simulink model "test_direct"  (R2024a)
settings: Solver=VariableStepAuto  StartTime=0.0  StopTime=40  RelTol=1e-3
libraries: neural x733, simulink x4
(part 25 of 35)

== system test_direct/Function Fitting Neural Network5/Layer 2/LW{2,1} ==
  "ad{2,1}" : Inport  PortDimensions=20
      mask Display: e = 0.06;c1 = [120 230 180]/255;c2 = ([120 230 180]+0)/(256+128);c3 = ([120 230 180]+128)/(256+128);patch([0 1 1 0],[0 0 1 1],c1);patch([0 1 1 1-e 1-e 0+e],[0 0 1 1-e 0+e 0+e],c2);patch([0 0 1 1-e 0+e 0+e],[0 1 1 1-e 1-e 0+e],c3);plot([0 1 1 0 0],[0 0 1 1 0]);
  "IW{2,1}(1,:)'" : Constant  Value=[-0.579046845479741278950314153917133808135986328125;-0.366332767141648307784862481639720499515533447265625;0.00791926397557877158328576427948064520023763179779052734375;0.355333435528304930617338186493725515902042388916015625;-0.19644275811117173358155696405447088181972503662109375;0.254735292145369107696950550234760157763957977294921875;0.36445816412065534795061694239848293364048004150390625;0.0304633669830193902494652746781866881065070629119873046875;0.74146026581714241654452735019731335341930389404296875;-0.0411865383465370438198505098625901155173778533935546875;0.10211270720633357222961734578348114155232906341552734375;0.1094855228463350871326298374697216786444187164306640625;1.093274183178303271546383257373236119747161865234375;-0.099686376669609499945323705105693079531192779541015625;-0.1438151389707562899378245901971240527927875518798828125;0.1476459310225679832928591395102557726204395294189453125;0.02646611700207172901411212251332472078502178192138671875;-0.42917127450968506341411057292134501039981842041015625;-0.184180448452047673679743411412346176803112030029296875;-0.0920595225436459940748790131692658178508281707763671875]
      mask Display: e = 0.06;c1 = [120 150 230]/255;c2 = ([120 150 230]+0)/383;c3 = ([120 150 230]+128)/383;patch([0 1 1 0],[0 0 1 1],c1);patch([0 1 1 1-e 1-e 0+e],[0 0 1 1-e 0+e 0+e],c2);patch([0 0 1 1-e 0+e 0+e],[0 1 1 1-e 1-e 0+e],c3);plot([0 1 1 0 0],[0 0 1 1 0]);disp('weights');
  "IW{2,1}(10,:)'" : Constant  Value=[0.45106523314206070640608459143550135195255279541015625;-0.006484688981325256902643605627645229105837643146514892578125;-0.600418159129877171409361835685558617115020751953125;0.59913844375957359122963907793746329843997955322265625;-0.76623092060152242499526664687437005341053009033203125;0.234260916721591883060682448558509349822998046875;0.7292760586627295982253826878149993717670440673828125;-0.449833710963811750360719088348560035228729248046875;0.3274752254953769980971856057294644415378570556640625;-0.47734563271799601569256310540367849171161651611328125;1.2532004567650962822966675958014093339443206787109375;-0.232482810204428125278042216450558044016361236572265625;-0.51335343850787673591895554636721499264240264892578125;0.01036668286886731869811395512215312919579446315765380859375;-0.0277386185034186084907847913427758612670004367828369140625;-0.049524443823777804241093036807797034271061420440673828125;0.02041516786832299479303998168688849546015262603759765625;0.013914717500251472248606887660571373999118804931640625;-0.041074885648775254221032326995555195026099681854248046875;-0.07560051804477367631829309857494081370532512664794921875]
      mask Display: e = 0.06;c1 = [120 150 230]/255;c2 = ([120 150 230]+0)/383;c3 = ([120 150 230]+128)/383;patch([0 1 1 0],[0 0 1 1],c1);patch([0 1 1 1-e 1-e 0+e],[0 0 1 1-e 0+e 0+e],c2);patch([0 0 1 1-e 0+e 0+e],[0 1 1 1-e 1-e 0+e],c3);plot([0 1 1 0 0],[0 0 1 1 0]);disp('weights');
  "IW{2,1}(2,:)'" : Constant  Value=[0.246046120338173024411076994510949589312076568603515625;-0.44416355549470665220468390543828718364238739013671875;-0.241828085176459761651557300865533761680126190185546875;0.048803101340167388821900118500707321800291538238525390625;0.2146749034455693594392045042695826850831508636474609375;-0.214628473377201867133834412015858106315135955810546875;0.304852751461086535211819636970176361501216888427734375;-0.26261872451235446224160341444076038897037506103515625;-0.37883423077533040501663208488025702536106109619140625;-0.262512916868190782082592704682610929012298583984375;-0.302067842690707577535391692435950972139835357666015625;-0.2059116523634101358908310430706478655338287353515625;0.277348751006312621569804832688532769680023193359375;-0.0667686637669950566742471664838376455008983612060546875;0.1551576203481833393649225172339356504380702972412109375;-0.156817869861261283137565669676405377686023712158203125;-0.64778006144449074010793765410198830068111419677734375;0.190002056867068558343447648439905606210231781005859375;0.3183559563991422702855516035924665629863739013671875;-0.65511604508801413171426020198850892484188079833984375]
      mask Display: e = 0.06;c1 = [120 150 230]/255;c2 = ([120 150 230]+0)/383;c3 = ([120 150 230]+128)/383;patch([0 1 1 0],[0 0 1 1],c1);patch([0 1 1 1-e 1-e 0+e],[0 0 1 1-e 0+e 0+e],c2);patch([0 0 1 1-e 0+e 0+e],[0 1 1 1-e 1-e 0+e],c3);plot([0 1 1 0 0],[0 0 1 1 0]);disp('weights');
  "IW{2,1}(3,:)'" : Constant  Value=[-0.352192261129181949375066551510826684534549713134765625;0.293665677168537087027289089746773242950439453125;-0.315518300729069889332123466374468989670276641845703125;-0.46790601172040224842163524954230524599552154541015625;0.0647169840392622652824883289213175885379314422607421875;-0.22641417805884866965016044559888541698455810546875;-0.421662956096390650895244789353455416858196258544921875;0.09447283223856751954716770569575601257383823394775390625;0.94313894621172511545381667019682936370372772216796875;0.182850302879195958372093855359707958996295928955078125;-0.2185526225368461805675934783721459098160266876220703125;-0.00908050016434655722641355879432012443430721759796142578125;0.7216056503661600896037953134509734809398651123046875;0.0604873719582102176151039429896627552807331085205078125;0.092237612451127104495895991931320168077945709228515625;-0.1472698116716875116338769657886587083339691162109375;0.0003899457974927842611283235196850682768854312598705291748046875;-0.071899880019338391345939953680499456822872161865234375;0.058786601922839187839286978487507440149784088134765625;0.07787533088066123099224569159559905529022216796875]
      mask Display: e = 0.06;c1 = [120 150 230]/255;c2 = ([120 150 230]+0)/383;c3 = ([120 150 230]+128)/383;patch([0 1 1 0],[0 0 1 1],c1);patch([0 1 1 1-e 1-e 0+e],[0 0 1 1-e 0+e 0+e],c2);patch([0 0 1 1-e 0+e 0+e],[0 1 1 1-e 1-e 0+e],c3);plot([0 1 1 0 0],[0 0 1 1 0]);disp('weights');
  "IW{2,1}(4,:)'" : Constant  Value=[-0.11038535014864879479912218585013761185109615325927734375;0.069052015333759708681782285566441714763641357421875;0.278344839855194148281469779249164275825023651123046875;-0.0429139321375657523116586844480480067431926727294921875;-0.14827093883976172339345112050068564713001251220703125;0.18100889775099648915102079627104103565216064453125;0.2070239482488422655404036731852102093398571014404296875;-0.1063017601653035992814722021648776717483997344970703125;-1.318163989884748144021386906388215720653533935546875;-0.098737455922967232169185081147588789463043212890625;0.214362322162434171257672232968616299331188201904296875;-0.03863337852201731426049491346930153667926788330078125;-0.588383198236690940774451519246213138103485107421875;-0.0272585835270687422415836209665940259583294391632080078125;0.000514366209257961369723244349216884074849076569080352783203125;0.054695929844052380841556981749818078242242336273193359375;-0.020553438564307725811008964456050307489931583404541015625;-0.468404405522319711163703459533280692994594573974609375;-0.02550599518226213946459068893091171048581600189208984375;-0.1348161547458721631898015402839519083499908447265625]
      mask Display: e = 0.06;c1 = [120 150 230]/255;c2 = ([120 150 230]+0)/383;c3 = ([120 150 230]+128)/383;patch([0 1 1 0],[0 0 1 1],c1);patch([0 1 1 1-e 1-e 0+e],[0 0 1 1-e 0+e 0+e],c2);patch([0 0 1 1-e 0+e 0+e],[0 1 1 1-e 1-e 0+e],c3);plot([0 1 1 0 0],[0 0 1 1 0]);disp('weights');
  "IW{2,1}(5,:)'" : Constant  Value=[0.7023428356000043226714524280396290123462677001953125;-0.184530133447649624667263879018719308078289031982421875;-0.1973243620284037824763601065569673664867877960205078125;0.352442802646694752777278836219920776784420013427734375;0.06548962322746569586495724024644005112349987030029296875;-0.538534813181375415780394178000278770923614501953125;0.027054454061479417392721558144330629147589206695556640625;0.4849622461151159580339253807323984801769256591796875;0.3562846230078176024136382693541236221790313720703125;0.2082065434670395120964059287871350534260272979736328125;0.647547883714221228501628502272069454193115234375;0.247394932810874268458434244166710413992404937744140625;-0.80148602251719880396052531068562529981136322021484375;0.0224490783621045415785477672443448682315647602081298828125;0.0869778231743936480757639628791366703808307647705078125;-0.2207666330910662277897671401660772971808910369873046875;-0.017685957506404927086496314814212382771074771881103515625;-0.34856979109160557417368409005575813353061676025390625;0.060254870992509833305117439294917858205735683441162109375;0.430945889886455102413265194627456367015838623046875]
      mask Display: e = 0.06;c1 = [120 150 230]/255;c2 = ([120 150 230]+0)/383;c3 = ([120 150 230]+128)/383;patch([0 1 1 0],[0 0 1 1],c1);patch([0 1 1 1-e 1-e 0+e],[0 0 1 1-e 0+e 0+e],c2);patch([0 0 1 1-e 0+e 0+e],[0 1 1 1-e 1-e 0+e],c3);plot([0 1 1 0 0],[0 0 1 1 0]);disp('weights');
  "IW{2,1}(6,:)'" : Constant  Value=[0.4224089115452738241174301947467029094696044921875;0.440056808161991386274536353084840811789035797119140625;-0.11419472374626714328282872656927793286740779876708984375;0.57575449411118595488545679472736082971096038818359375;-0.2331470229256961401720360527178854681551456451416015625;-0.423016524638085422704847360364510677754878997802734375;1.363489995339575155952616114518605172634124755859375;-1.0868187458133322653708319194265641272068023681640625;-0.10913236701853497312431073851257679052650928497314453125;0.799982620513981945720161093049682676792144775390625;-0.182307650456612180267512712816824205219745635986328125;0.37545487088480145043689617523341439664363861083984375;0.41570000943437579454808883383520878851413726806640625;0.023541045860106489528984496928387670777738094329833984375;0.473684260454336258927554581532604061067104339599609375;1.2657571479447373707927226860192604362964630126953125;-0.1829983548740201637627933450858108699321746826171875;-0.221247927654384113349550489147077314555644989013671875;-0.367143898363431142595203482414945028722286224365234375;0.0019581555874889507683211942179468678659759461879730224609375]
      mask Display: e = 0.06;c1 = [120 150 230]/255;c2 = ([120 150 230]+0)/383;c3 = ([120 150 230]+128)/383;patch([0 1 1 0],[0 0 1 1],c1);patch([0 1 1 1-e 1-e 0+e],[0 0 1 1-e 0+e 0+e],c2);patch([0 0 1 1-e 0+e 0+e],[0 1 1 1-e 1-e 0+e],c3);plot([0 1 1 0 0],[0 0 1 1 0]);disp('weights');
  "IW{2,1}(7,:)'" : Constant  Value=[0.85279025027125465729938014192157424986362457275390625;0.08683805962927020061226102143336902372539043426513671875;-0.1673040176973877024568793103753705509006977081298828125;0.184731321925173885833970643943757750093936920166015625;0.7682354316165156404849767568521201610565185546875;-0.1796643086082986007223638580398983322083950042724609375;0.521167175396772375250975528615526854991912841796875;0.297359432301631476658343444796628318727016448974609375;0.99940927153345715527876791384187527000904083251953125;-0.4141002194910043954223510809242725372314453125;0.277484240839730500471915775051456876099109649658203125;0.3502208837605882418841929393238388001918792724609375;-0.51455921650667202360551755191409029066562652587890625;-0.022741456932024471659925524136269814334809780120849609375;0.270467721739372113365362793047097511589527130126953125;-0.08357141079773365566207843357915407977998256683349609375;-0.1332513992108804445901881763347773812711238861083984375;0.0696241608697020508689234929988742806017398834228515625;0.311943119438749472127625494977110065519809722900390625;-0.032764834535114299718383534809618140570819377899169921875]
      mask Display: e = 0.06;c1 = [120 150 230]/255;c2 = ([120 150 230]+0)/383;c3 = ([120 150 230]+128)/383;patch([0 1 1 0],[0 0 1 1],c1);patch([0 1 1 1-e 1-e 0+e],[0 0 1 1-e 0+e 0+e],c2);patch([0 0 1 1-e 0+e 0+e],[0 1 1 1-e 1-e 0+e],c3);plot([0 1 1 0 0],[0 0 1 1 0]);disp('weights');
  "IW{2,1}(8,:)'" : Constant  Value=[0.498452840354915716059025498907431028783321380615234375;0.366558574940812842424264772489550523459911346435546875;-0.1510456402745621318217672524042427539825439453125;-0.0769269745328168552678249625387252308428287506103515625;0.3004215881244201025168649721308611333370208740234375;-0.490819816489340199350266402689157985150814056396484375;0.1364661808556923150437256708755739964544773101806640625;0.384791567617603524897873512600199319422245025634765625;0.7867187025807071965033401284017600119113922119140625;-0.6146433979166905370306039912975393235683441162109375;0.497314382965974022265953635724144987761974334716796875;-0.08779484862380086684918722994552808813750743865966796875;-0.08995292924666446754411452957356232218444347381591796875;-0.07126163880156348440220170914471964351832866668701171875;-0.756117230801268913609192168223671615123748779296875;0.0225922316589895998129033927170894457958638668060302734375;0.313500674283847702294991677263169549405574798583984375;0.11989233760044448739989775276626460254192352294921875;-0.18563408446150686526010531451902352273464202880859375;-0.050881810495495095880702507429305114783346652984619140625]
      mask Display: e = 0.06;c1 = [120 150 230]/255;c2 = ([120 150 230]+0)/383;c3 = ([120 150 230]+128)/383;patch([0 1 1 0],[0 0 1 1],c1);patch([0 1 1 1-e 1-e 0+e],[0 0 1 1-e 0+e 0+e],c2);patch([0 0 1 1-e 0+e 0+e],[0 1 1 1-e 1-e 0+e],c3);plot([0 1 1 0 0],[0 0 1 1 0]);disp('weights');
  "IW{2,1}(9,:)'" : Constant  Value=[0.290579186072249751049412225256673991680145263671875;0.366662252183763082147294198875897563993930816650390625;0.1440875193407215870688986569803091697394847869873046875;-0.0302403581180806131645244505534719792194664478302001953125;0.100950277691890966114129923880682326853275299072265625;0.1381393716982420583061497154631069861352443695068359375;0.331727150444919127725285079577588476240634918212890625;-0.4425342659789885946253207293921150267124176025390625;-0.023796097376492665598224363066037767566740512847900390625;0.25120426572081366867195129088941030204296112060546875;-0.287894666419527600620398288810974918305873870849609375;-0.157619878708374294706828777634655125439167022705078125;-0.6348198907290776293876888303202576935291290283203125;0.10107959034423912025868474984235945157706737518310546875;0.6616827948368395606593139746109955012798309326171875;-0.487640617460125491700040356590761803090572357177734375;-0.380966735137811596256796065063099376857280731201171875;0.1969944624768071583797990342645789496600627899169921875;0.491439123097786201288528218356077559292316436767578125;-0.481116141212482417710560866908053867518901824951171875]
      mask Display: e = 0.06;c1 = [120 150 230]/255;c2 = ([120 150 230]+0)/383;c3 = ([120 150 230]+128)/383;patch([0 1 1 0],[0 0 1 1],c1);patch([0 1 1 1-e 1-e 0+e],[0 0 1 1-e 0+e 0+e],c2);patch([0 0 1 1-e 0+e 0+e],[0 1 1 1-e 1-e 0+e],c3);plot([0 1 1 0 0],[0 0 1 1 0]);disp('weights');
  Mux : Mux  Inputs=10
      mask Display: e = 0.06;c1 = [120 150 230]/255;c2 = ([120 150 230]+0)/383;c3 = ([120 150 230]+128)/383;patch([0 1 1 0],[0 0 1 1],c1);patch([0 1 1 1-e 1-e 0+e],[0 0 1 1-e 0+e 0+e],c2);patch([0 0 1 1-e 0+e 0+e],[0 1 1 1-e 1-e 0+e],c3);plot([0 1 1 0 0],[0 0 1 1 0]);disp('Mux');
  dotprod{1..10} (10 alike) : neural/Weight Functions/dotprod
  "lz{2,1}" : Outport
      mask Display: e = 0.06;c1 = [120 230 180]/255;c2 = ([120 230 180]+0)/(256+128);c3 = ([120 230 180]+128)/(256+128);patch([0 1 1 0],[0 0 1 1],c1);patch([0 1 1 1-e 1-e 0+e],[0 0 1 1-e 0+e 0+e],c2);patch([0 0 1 1-e 0+e 0+e],[0 1 1 1-e 1-e 0+e],c3);plot([0 1 1 0 0],[0 0 1 1 0]);
  wires:
  "IW{2,1}(1,:)'"/1 -> dotprod1/1
  "ad{2,1}"/1 -> dotprod1/2, dotprod2/2, dotprod3/2, dotprod4/2, dotprod5/2, dotprod6/2, dotprod7/2, dotprod8/2, dotprod9/2, dotprod10/2
  dotprod1/1 -> Mux/1
  "IW{2,1}(2,:)'"/1 -> dotprod2/1
  dotprod2/1 -> Mux/2
  "IW{2,1}(3,:)'"/1 -> dotprod3/1
  dotprod3/1 -> Mux/3
  "IW{2,1}(4,:)'"/1 -> dotprod4/1
  dotprod4/1 -> Mux/4
  "IW{2,1}(5,:)'"/1 -> dotprod5/1
  dotprod5/1 -> Mux/5
  "IW{2,1}(6,:)'"/1 -> dotprod6/1
  dotprod6/1 -> Mux/6
  "IW{2,1}(7,:)'"/1 -> dotprod7/1
  dotprod7/1 -> Mux/7
  "IW{2,1}(8,:)'"/1 -> dotprod8/1
  dotprod8/1 -> Mux/8
  "IW{2,1}(9,:)'"/1 -> dotprod9/1
  dotprod9/1 -> Mux/9
  "IW{2,1}(10,:)'"/1 -> dotprod10/1
  dotprod10/1 -> Mux/10
  Mux/1 -> "lz{2,1}"/1

== system test_direct/Function Fitting Neural Network5/Layer 3/Delays 1 ==
  "p{3}" : Inport  PortDimensions=10
      mask Display: e = 0.06;c1 = [120 230 180]/255;c2 = ([120 230 180]+0)/(256+128);c3 = ([120 230 180]+128)/(256+128);patch([0 1 1 0],[0 0 1 1],c1);patch([0 1 1 1-e 1-e 0+e],[0 0 1 1-e 0+e 0+e],c2);patch([0 0 1 1-e 0+e 0+e],[0 1 1 1-e 1-e 0+e],c3);plot([0 1 1 0 0],[0 0 1 1 0]);
  mux : Mux  Inputs=1
      mask Display: e = 0.06;c1 = [120 150 230]/255;c2 = ([120 150 230]+0)/383;c3 = ([120 150 230]+128)/383;patch([0 1 1 0],[0 0 1 1],c1);patch([0 1 1 1-e 1-e 0+e],[0 0 1 1-e 0+e 0+e],c2);patch([0 0 1 1-e 0+e 0+e],[0 1 1 1-e 1-e 0+e],c3);plot([0 1 1 0 0],[0 0 1 1 0]);disp('Mux')
  "pd{3,2}" : Outport
      mask Display: e = 0.06;c1 = [120 230 180]/255;c2 = ([120 230 180]+0)/(256+128);c3 = ([120 230 180]+128)/(256+128);patch([0 1 1 0],[0 0 1 1],c1);patch([0 1 1 1-e 1-e 0+e],[0 0 1 1-e 0+e 0+e],c2);patch([0 0 1 1-e 0+e 0+e],[0 1 1 1-e 1-e 0+e],c3);plot([0 1 1 0 0],[0 0 1 1 0]);
  wires:
  "p{3}"/1 -> mux/1
  mux/1 -> "pd{3,2}"/1

== system test_direct/Function Fitting Neural Network5/Layer 3/LW{3,2} ==
  "ad{3,2}" : Inport  PortDimensions=10
      mask Display: e = 0.06;c1 = [120 230 180]/255;c2 = ([120 230 180]+0)/(256+128);c3 = ([120 230 180]+128)/(256+128);patch([0 1 1 0],[0 0 1 1],c1);patch([0 1 1 1-e 1-e 0+e],[0 0 1 1-e 0+e 0+e],c2);patch([0 0 1 1-e 0+e 0+e],[0 1 1 1-e 1-e 0+e],c3);plot([0 1 1 0 0],[0 0 1 1 0]);
  "IW{3,2}(1,:)'" : Constant  Value=[0.79370873300215050161199314970872364938259124755859375;-0.3200226311081910690603535840637050569057464599609375;1.2061996125942109348017083902959711849689483642578125;-1.5615997523335156671464574174024164676666259765625;-0.75490200592473011287353301668190397322177886962890625;-0.11063883079028712097535702696404769085347652435302734375;0.5845904369092311814171125661232508718967437744140625;0.04601777779405673285406663808316807262599468231201171875;-0.7115838685892506010333136146073229610919952392578125;-0.5017512522185627599213830762892030179500579833984375]
      mask Display: e = 0.06;c1 = [120 150 230]/255;c2 = ([120 150 230]+0)/383;c3 = ([120 150 230]+128)/383;patch([0 1 1 0],[0 0 1 1],c1);patch([0 1 1 1-e 1-e 0+e],[0 0 1 1-e 0+e 0+e],c2);patch([0 0 1 1-e 0+e 0+e],[0 1 1 1-e 1-e 0+e],c3);plot([0 1 1 0 0],[0 0 1 1 0]);disp('weights');
  "IW{3,2}(2,:)'" : Constant  Value=[-0.28960166204355208829923640223569236695766448974609375;-0.0252574701415183740238479259687665035016834735870361328125;-0.0958925927891242924072656705902772955596446990966796875;0.06445536465388544689059102665851241908967494964599609375;0.2594143192737743408571304826182313263416290283203125;0.16773287966872107990212725781020708382129669189453125;0.73734001878716337596841867707553319633007049560546875;0.10779251526925580362270551404435536824166774749755859375;0.03260513731556773098230195273572462610900402069091796875;0.97907124259663103060802313848398625850677490234375]
      mask Display: e = 0.06;c1 = [120 150 230]/255;c2 = ([120 150 230]+0)/383;c3 = ([120 150 230]+128)/383;patch([0 1 1 0],[0 0 1 1],c1);patch([0 1 1 1-e 1-e 0+e],[0 0 1 1-e 0+e 0+e],c2);patch([0 0 1 1-e 0+e 0+e],[0 1 1 1-e 1-e 0+e],c3);plot([0 1 1 0 0],[0 0 1 1 0]);disp('weights');
  Mux : Mux  Inputs=2
      mask Display: e = 0.06;c1 = [120 150 230]/255;c2 = ([120 150 230]+0)/383;c3 = ([120 150 230]+128)/383;patch([0 1 1 0],[0 0 1 1],c1);patch([0 1 1 1-e 1-e 0+e],[0 0 1 1-e 0+e 0+e],c2);patch([0 0 1 1-e 0+e 0+e],[0 1 1 1-e 1-e 0+e],c3);plot([0 1 1 0 0],[0 0 1 1 0]);disp('Mux');
  dotprod1 : neural/Weight Functions/dotprod
  dotprod2 : neural/Weight Functions/dotprod
  "lz{3,2}" : Outport
      mask Display: e = 0.06;c1 = [120 230 180]/255;c2 = ([120 230 180]+0)/(256+128);c3 = ([120 230 180]+128)/(256+128);patch([0 1 1 0],[0 0 1 1],c1);patch([0 1 1 1-e 1-e 0+e],[0 0 1 1-e 0+e 0+e],c2);patch([0 0 1 1-e 0+e 0+e],[0 1 1 1-e 1-e 0+e],c3);plot([0 1 1 0 0],[0 0 1 1 0]);
  wires:
  "IW{3,2}(1,:)'"/1 -> dotprod1/1
  "ad{3,2}"/1 -> dotprod1/2, dotprod2/2
  dotprod1/1 -> Mux/1
  "IW{3,2}(2,:)'"/1 -> dotprod2/1
  dotprod2/1 -> Mux/2
  Mux/1 -> "lz{3,2}"/1

== system test_direct/Function Fitting Neural Network6/Layer 1/Delays 1 ==
  "p{1}" : Inport  PortDimensions=8
      mask Display: e = 0.06;c1 = [120 230 180]/255;c2 = ([120 230 180]+0)/(256+128);c3 = ([120 230 180]+128)/(256+128);patch([0 1 1 0],[0 0 1 1],c1);patch([0 1 1 1-e 1-e 0+e],[0 0 1 1-e 0+e 0+e],c2);patch([0 0 1 1-e 0+e 0+e],[0 1 1 1-e 1-e 0+e],c3);plot([0 1 1 0 0],[0 0 1 1 0]);
  mux : Mux  Inputs=1
      mask Display: e = 0.06;c1 = [120 150 230]/255;c2 = ([120 150 230]+0)/383;c3 = ([120 150 230]+128)/383;patch([0 1 1 0],[0 0 1 1],c1);patch([0 1 1 1-e 1-e 0+e],[0 0 1 1-e 0+e 0+e],c2);patch([0 0 1 1-e 0+e 0+e],[0 1 1 1-e 1-e 0+e],c3);plot([0 1 1 0 0],[0 0 1 1 0]);disp('Mux')
  "pd{1,1}" : Outport
      mask Display: e = 0.06;c1 = [120 230 180]/255;c2 = ([120 230 180]+0)/(256+128);c3 = ([120 230 180]+128)/(256+128);patch([0 1 1 0],[0 0 1 1],c1);patch([0 1 1 1-e 1-e 0+e],[0 0 1 1-e 0+e 0+e],c2);patch([0 0 1 1-e 0+e 0+e],[0 1 1 1-e 1-e 0+e],c3);plot([0 1 1 0 0],[0 0 1 1 0]);
  wires:
  "p{1}"/1 -> mux/1
  mux/1 -> "pd{1,1}"/1

== system test_direct/Function Fitting Neural Network6/Layer 1/IW{1,1} ==
  "pd{1,1}" : Inport  PortDimensions=8
      mask Display: e = 0.06;c1 = [120 230 180]/255;c2 = ([120 230 180]+0)/(256+128);c3 = ([120 230 180]+128)/(256+128);patch([0 1 1 0],[0 0 1 1],c1);patch([0 1 1 1-e 1-e 0+e],[0 0 1 1-e 0+e 0+e],c2);patch([0 0 1 1-e 0+e 0+e],[0 1 1 1-e 1-e 0+e],c3);plot([0 1 1 0 0],[0 0 1 1 0]);
  "IW{1,1}(1,:)'" : Constant  Value=[0.23210165099576063330033548481878824532032012939453125;0.40383818649639213749225064020720310509204864501953125;0.79204303168135592461140959130716510117053985595703125;-0.68445510326316227889265064732171595096588134765625;0.004580398428411481918931524859317505615763366222381591796875;-0.36059519966918396338684260626905597746372222900390625;-0.7280780112290334837865657391375862061977386474609375;0.85155447541191120475190245997509919106960296630859375]
      mask Display: e = 0.06;c1 = [120 150 230]/255;c2 = ([120 150 230]+0)/383;c3 = ([120 150 230]+128)/383;patch([0 1 1 0],[0 0 1 1],c1);patch([0 1 1 1-e 1-e 0+e],[0 0 1 1-e 0+e 0+e],c2);patch([0 0 1 1-e 0+e 0+e],[0 1 1 1-e 1-e 0+e],c3);plot([0 1 1 0 0],[0 0 1 1 0]);disp('Weights');
  "IW{1,1}(10,:)'" : Constant  Value=[0.038689906436106931419960375251321238465607166290283203125;0.1047931051610293540221618968644179403781890869140625;0.2421340157351225264026339800693676806986331939697265625;-0.0184510120990238508931202687790573691017925739288330078125;-0.382830714590992660095736255243537016212940216064453125;1.103210523666664499842227087356150150299072265625;-0.1295286959930661840889598579451558180153369903564453125;-1.2567031084613227154278547459398396313190460205078125]
      mask Display: e = 0.06;c1 = [120 150 230]/255;c2 = ([120 150 230]+0)/383;c3 = ([120 150 230]+128)/383;patch([0 1 1 0],[0 0 1 1],c1);patch([0 1 1 1-e 1-e 0+e],[0 0 1 1-e 0+e 0+e],c2);patch([0 0 1 1-e 0+e 0+e],[0 1 1 1-e 1-e 0+e],c3);plot([0 1 1 0 0],[0 0 1 1 0]);disp('Weights');
  "IW{1,1}(11,:)'" : Constant  Value=[0.38094161831417705510460791629157029092311859130859375;-0.3872849190639058303275987782399170100688934326171875;0.63596921647638826602388917308417148888111114501953125;0.601401314142957943431611056439578533172607421875;-0.91288468798632649292557061926345340907573699951171875;0.07028815046685378542523636724581592716276645660400390625;0.78751934238677068211842424716451205313205718994140625;0.266681940054065147460704565673950128257274627685546875]
      mask Display: e = 0.06;c1 = [120 150 230]/255;c2 = ([120 150 230]+0)/383;c3 = ([120 150 230]+128)/383;patch([0 1 1 0],[0 0 1 1],c1);patch([0 1 1 1-e 1-e 0+e],[0 0 1 1-e 0+e 0+e],c2);patch([0 0 1 1-e 0+e 0+e],[0 1 1 1-e 1-e 0+e],c3);plot([0 1 1 0 0],[0 0 1 1 0]);disp('Weights');
  "IW{1,1}(12,:)'" : Constant  Value=[-0.20687419587863609127253994302009232342243194580078125;0.344885104461707336920284205916686914861202239990234375;-0.01424083408136080954042856916430537239648401737213134765625;0.4791958882549953724350189077085815370082855224609375;0.06143452087041893772134670825835200957953929901123046875;0.79895991503677687983753230582806281745433807373046875;1.087157101682284743304762741900049149990081787109375;-0.193819992190888801264492258269456215202808380126953125]
      mask Display: e = 0.06;c1 = [120 150 230]/255;c2 = ([120 150 230]+0)/383;c3 = ([120 150 230]+128)/383;patch([0 1 1 0],[0 0 1 1],c1);patch([0 1 1 1-e 1-e 0+e],[0 0 1 1-e 0+e 0+e],c2);patch([0 0 1 1-e 0+e 0+e],[0 1 1 1-e 1-e 0+e],c3);plot([0 1 1 0 0],[0 0 1 1 0]);disp('Weights');
  "IW{1,1}(13,:)'" : Constant  Value=[0.16172124765613882235726350700133480131626129150390625;0.1488452757625824685039361838789773173630237579345703125;-0.299942382464043644230144991524866782128810882568359375;-0.7930426482578949443080773562542162835597991943359375;-0.03286265064662775847725839639679179526865482330322265625;-0.95035904961144190838950862598721869289875030517578125;-0.86651027713978567845742873032577335834503173828125;-0.026111279232306362774185259922887780703604221343994140625]
      mask Display: e = 0.06;c1 = [120 150 230]/255;c2 = ([120 150 230]+0)/383;c3 = ([120 150 230]+128)/383;patch([0 1 1 0],[0 0 1 1],c1);patch([0 1 1 1-e 1-e 0+e],[0 0 1 1-e 0+e 0+e],c2);patch([0 0 1 1-e 0+e 0+e],[0 1 1 1-e 1-e 0+e],c3);plot([0 1 1 0 0],[0 0 1 1 0]);disp('Weights');
  "IW{1,1}(14,:)'" : Constant  Value=[0.3288914029355527457454400064307264983654022216796875;-0.26053858625059411746605064763571135699748992919921875;0.50567878034036317647093028426752425730228424072265625;0.33909664239978687394483358730212785303592681884765625;0.33806965806520938855328495264984667301177978515625;-0.7487601196664452896101238366100005805492401123046875;-0.381097160006196478132522997839259915053844451904296875;1.1162819026891324103445413129520602524280548095703125]
      mask Display: e = 0.06;c1 = [120 150 230]/255;c2 = ([120 150 230]+0)/383;c3 = ([120 150 230]+128)/383;patch([0 1 1 0],[0 0 1 1],c1);patch([0 1 1 1-e 1-e 0+e],[0 0 1 1-e 0+e 0+e],c2);patch([0 0 1 1-e 0+e 0+e],[0 1 1 1-e 1-e 0+e],c3);plot([0 1 1 0 0],[0 0 1 1 0]);disp('Weights');
  "IW{1,1}(15,:)'" : Constant  Value=[0.01516380106283477836870421384674045839346945285797119140625;-0.08414140469319843218531929096570820547640323638916015625;-0.06705189830474200807230999998864717781543731689453125;0.1358539930663603401139738480196683667600154876708984375;1.1857362963726101323658213004819117486476898193359375;0.2007411467744188160455820479910471476614475250244140625;-1.4364253304956358103794400449260137975215911865234375;-0.9112373448160797639872043873765505850315093994140625]
      mask Display: e = 0.06;c1 = [120 150 230]/255;c2 = ([120 150 230]+0)/383;c3 = ([120 150 230]+128)/383;patch([0 1 1 0],[0 0 1 1],c1);patch([0 1 1 1-e 1-e 0+e],[0 0 1 1-e 0+e 0+e],c2);patch([0 0 1 1-e 0+e 0+e],[0 1 1 1-e 1-e 0+e],c3);plot([0 1 1 0 0],[0 0 1 1 0]);disp('Weights');
  "IW{1,1}(16,:)'" : Constant  Value=[-0.52244152315840508560285115891019813716411590576171875;-0.233975539497325246696135536694782786071300506591796875;0.1867457360834435531327102353316149674355983734130859375;0.05021332645405528205539980035609914921224117279052734375;-0.5316371447247860704266031461884267628192901611328125;0.7204185510281515547603703453205525875091552734375;-0.82954581048569242529566736266133375465869903564453125;0.0109751016767199345569583357473675278015434741973876953125]
      mask Display: e = 0.06;c1 = [120 150 230]/255;c2 = ([120 150 230]+0)/383;c3 = ([120 150 230]+128)/383;patch([0 1 1 0],[0 0 1 1],c1);patch([0 1 1 1-e 1-e 0+e],[0 0 1 1-e 0+e 0+e],c2);patch([0 0 1 1-e 0+e 0+e],[0 1 1 1-e 1-e 0+e],c3);plot([0 1 1 0 0],[0 0 1 1 0]);disp('Weights');
  "IW{1,1}(17,:)'" : Constant  Value=[-0.039427549023366613434316008124369545839726924896240234375;0.04958542310555920373804639211812173016369342803955078125;-0.324273606753851806328015072722337208688259124755859375;0.9563591423617416875657681885058991611003875732421875;0.9770784355523767228390852324082516133785247802734375;-0.5552235063018022831471398603753186762332916259765625;0.60891129045042158285383493421250022947788238525390625;-0.5170697194429030307816219647065736353397369384765625]
      mask Display: e = 0.06;c1 = [120 150 230]/255;c2 = ([120 150 230]+0)/383;c3 = ([120 150 230]+128)/383;patch([0 1 1 0],[0 0 1 1],c1);patch([0 1 1 1-e 1-e 0+e],[0 0 1 1-e 0+e 0+e],c2);patch([0 0 1 1-e 0+e 0+e],[0 1 1 1-e 1-e 0+e],c3);plot([0 1 1 0 0],[0 0 1 1 0]);disp('Weights');
  "IW{1,1}(18,:)'" : Constant  Value=[0.061158393864709927056910743203843594528734683990478515625;0.62352759942049740260472390218637883663177490234375;0.259189784391532451746087417632224969565868377685546875;-0.60149527059616081370307938414043746888637542724609375;0.4926650151859417459121459614834748208522796630859375;0.58476803055227166705520858158706687390804290771484375;-0.032815685249065272566237894125151797197759151458740234375;1.0579329581221694756010265336954034864902496337890625]
      mask Display: e = 0.06;c1 = [120 150 230]/255;c2 = ([120 150 230]+0)/383;c3 = ([120 150 230]+128)/383;patch([0 1 1 0],[0 0 1 1],c1);patch([0 1 1 1-e 1-e 0+e],[0 0 1 1-e 0+e 0+e],c2);patch([0 0 1 1-e 0+e 0+e],[0 1 1 1-e 1-e 0+e],c3);plot([0 1 1 0 0],[0 0 1 1 0]);disp('Weights');
  "IW{1,1}(19,:)'" : Constant  Value=[0.32970113319397753581796450816909782588481903076171875;-0.7982797504075451744398606024333275854587554931640625;-0.07813437768007690242821894344160682521760463714599609375;-0.42604131584556370615501919019152410328388214111328125;0.6674352103600387220438960866886191070079803466796875;0.738899057975787254548549753963015973567962646484375;-0.46073841260685977072597552250954322516918182373046875;-1.039989031819163134429118144907988607883453369140625]
      mask Display: e = 0.06;c1 = [120 150 230]/255;c2 = ([120 150 230]+0)/383;c3 = ([120 150 230]+128)/383;patch([0 1 1 0],[0 0 1 1],c1);patch([0 1 1 1-e 1-e 0+e],[0 0 1 1-e 0+e 0+e],c2);patch([0 0 1 1-e 0+e 0+e],[0 1 1 1-e 1-e 0+e],c3);plot([0 1 1 0 0],[0 0 1 1 0]);disp('Weights');
  "IW{1,1}(2,:)'" : Constant  Value=[-0.57708662632656793078922419226728379726409912109375;0.371853602206976052713116587256081402301788330078125;0.7999846505363166215829551219940185546875;0.999671612818497035135578698827885091304779052734375;-0.433111624096211345058549113673507235944271087646484375;-0.826422974445387037434329613461159169673919677734375;-0.0033898901654064749790207233814953724504448473453521728515625;-0.455639717919369247045580095800687558948993682861328125]
      mask Display: e = 0.06;c1 = [120 150 230]/255;c2 = ([120 150 230]+0)/383;c3 = ([120 150 230]+128)/383;patch([0 1 1 0],[0 0 1 1],c1);patch([0 1 1 1-e 1-e 0+e],[0 0 1 1-e 0+e 0+e],c2);patch([0 0 1 1-e 0+e 0+e],[0 1 1 1-e 1-e 0+e],c3);plot([0 1 1 0 0],[0 0 1 1 0]);disp('Weights');
  "IW{1,1}(20,:)'" : Constant  Value=[0.2010385837184836266278153971143183298408985137939453125;-0.24473039286824349591853433594224043190479278564453125;-0.60984506709114272293703606919734738767147064208984375;0.038143520332834822406109509529414935968816280364990234375;-0.98931750236619186988917817870969884097576141357421875;1.348284521851762729482970826211385428905487060546875;-0.11962768857278739675908951767269172705709934234619140625;-0.2188188737634802760734231696915230713784694671630859375]
      mask Display: e = 0.06;c1 = [120 150 230]/255;c2 = ([120 150 230]+0)/383;c3 = ([120 150 230]+128)/383;patch([0 1 1 0],[0 0 1 1],c1);patch([0 1 1 1-e 1-e 0+e],[0 0 1 1-e 0+e 0+e],c2);patch([0 0 1 1-e 0+e 0+e],[0 1 1 1-e 1-e 0+e],c3);plot([0 1 1 0 0],[0 0 1 1 0]);disp('Weights');
  "IW{1,1}(3,:)'" : Constant  Value=[0.1316678118764886828984117528307251632213592529296875;-0.3743871351267908931248484805109910666942596435546875;-0.6883020925337619555506307733594439923763275146484375;0.54749093036277474144668531153001822531223297119140625;0.198387999873663234406961919376044534146785736083984375;-0.52958253926801213129493817177717573940753936767578125;-1.0671153067001208913922027932130731642246246337890625;-0.9224385014164173668405055650509893894195556640625]
      mask Display: e = 0.06;c1 = [120 150 230]/255;c2 = ([120 150 230]+0)/383;c3 = ([120 150 230]+128)/383;patch([0 1 1 0],[0 0 1 1],c1);patch([0 1 1 1-e 1-e 0+e],[0 0 1 1-e 0+e 0+e],c2);patch([0 0 1 1-e 0+e 0+e],[0 1 1 1-e 1-e 0+e],c3);plot([0 1 1 0 0],[0 0 1 1 0]);disp('Weights');
  "IW{1,1}(4,:)'" : Constant  Value=[0.52090425064992895709536924186977557837963104248046875;-0.1416445301208219265109988782569416798651218414306640625;-0.5968854147969369083881474580266512930393218994140625;0.9217354460530688964325918277609162032604217529296875;-0.704143835761208425338963934336788952350616455078125;0.57164535424231821547635945535148493945598602294921875;0.10958559524149975861195827064875629730522632598876953125;-0.806130485552817521721635785070247948169708251953125]
      mask Display: e = 0.06;c1 = [120 150 230]/255;c2 = ([120 150 230]+0)/383;c3 = ([120 150 230]+128)/383;patch([0 1 1 0],[0 0 1 1],c1);patch([0 1 1 1-e 1-e 0+e],[0 0 1 1-e 0+e 0+e],c2);patch([0 0 1 1-e 0+e 0+e],[0 1 1 1-e 1-e 0+e],c3);plot([0 1 1 0 0],[0 0 1 1 0]);disp('Weights');
  "IW{1,1}(5,:)'" : Constant  Value=[-0.168024156978862693190279742339043878018856048583984375;-0.10820794686916757054717663777410052716732025146484375;0.059989101690901831809288324848239426501095294952392578125;0.77346004662645995164638179630856029689311981201171875;0.06687957865994124950770327586724306456744670867919921875;-0.41941981592018284796807847669697366654872894287109375;-0.6241252311504876804093555620056577026844024658203125;1.270030496885986348587493921513669192790985107421875]
      mask Display: e = 0.06;c1 = [120 150 230]/255;c2 = ([120 150 230]+0)/383;c3 = ([120 150 230]+128)/383;patch([0 1 1 0],[0 0 1 1],c1);patch([0 1 1 1-e 1-e 0+e],[0 0 1 1-e 0+e 0+e],c2);patch([0 0 1 1-e 0+e 0+e],[0 1 1 1-e 1-e 0+e],c3);plot([0 1 1 0 0],[0 0 1 1 0]);disp('Weights');
  "IW{1,1}(6,:)'" : Constant  Value=[-0.1078650523035900310464541007604566402733325958251953125;-0.3955893898582363288340957296895794570446014404296875;0.4413780485409939391416855869465507566928863525390625;-0.05052207368383605790018719972067628987133502960205078125;1.003837082235297106791449550655670464038848876953125;0.9123244326099555490117154477047733962535858154296875;-0.77469282341323353335837964550592005252838134765625;0.70938009131881474278458199478336609899997711181640625]
      mask Display: e = 0.06;c1 = [120 150 230]/255;c2 = ([120 150 230]+0)/383;c3 = ([120 150 230]+128)/383;patch([0 1 1 0],[0 0 1 1],c1);patch([0 1 1 1-e 1-e 0+e],[0 0 1 1-e 0+e 0+e],c2);patch([0 0 1 1-e 0+e 0+e],[0 1 1 1-e 1-e 0+e],c3);plot([0 1 1 0 0],[0 0 1 1 0]);disp('Weights');
  "IW{1,1}(7,:)'" : Constant  Value=[-0.0764940311798422423184007357122027315199375152587890625;0.184512546969679391839491700011421926319599151611328125;0.62735229395625446979778416789486072957515716552734375;-0.2582953928434588153351114669931121170520782470703125;-0.2252491234735270742017831935299909673631191253662109375;0.00015404363538832339225979894958840077379136346280574798583984375;-0.9005426658149355834126481568091548979282379150390625;0.6369533758721390714896415374823845922946929931640625]
      mask Display: e = 0.06;c1 = [120 150 230]/255;c2 = ([120 150 230]+0)/383;c3 = ([120 150 230]+128)/383;patch([0 1 1 0],[0 0 1 1],c1);patch([0 1 1 1-e 1-e 0+e],[0 0 1 1-e 0+e 0+e],c2);patch([0 0 1 1-e 0+e 0+e],[0 1 1 1-e 1-e 0+e],c3);plot([0 1 1 0 0],[0 0 1 1 0]);disp('Weights');
  "IW{1,1}(8,:)'" : Constant  Value=[0.1419593257168541844404074936392134986817836761474609375;-0.1048502611523287886274857783064362592995166778564453125;-0.325610064311064262287942483453662134706974029541015625;0.129747796763379719120479194316430948674678802490234375;0.52113541293190468461915543230134062469005584716796875;-0.6743567847221376698740868960157968103885650634765625;-1.0099409127016034659618526347912847995758056640625;1.08986325192531641192772440263070166110992431640625]
      mask Display: e = 0.06;c1 = [120 150 230]/255;c2 = ([120 150 230]+0)/383;c3 = ([120 150 230]+128)/383;patch([0 1 1 0],[0 0 1 1],c1);patch([0 1 1 1-e 1-e 0+e],[0 0 1 1-e 0+e 0+e],c2);patch([0 0 1 1-e 0+e 0+e],[0 1 1 1-e 1-e 0+e],c3);plot([0 1 1 0 0],[0 0 1 1 0]);disp('Weights');
  "IW{1,1}(9,:)'" : Constant  Value=[-0.191192052700136005949360651356982998549938201904296875;-0.48761277828526294886302139275358058512210845947265625;0.68077556166938613113615019756252877414226531982421875;-0.356155172923465268564058305855724029242992401123046875;0.424529467101340041157442328767501749098300933837890625;-0.414148460413097552201833195795188657939434051513671875;0.5783532579379393467888803570531308650970458984375;0.70285200171775052968570207667653448879718780517578125]
      mask Display: e = 0.06;c1 = [120 150 230]/255;c2 = ([120 150 230]+0)/383;c3 = ([120 150 230]+128)/383;patch([0 1 1 0],[0 0 1 1],c1);patch([0 1 1 1-e 1-e 0+e],[0 0 1 1-e 0+e 0+e],c2);patch([0 0 1 1-e 0+e 0+e],[0 1 1 1-e 1-e 0+e],c3);plot([0 1 1 0 0],[0 0 1 1 0]);disp('Weights');
  Mux : Mux  Inputs=20
      mask Display: e = 0.06;c1 = [120 150 230]/255;c2 = ([120 150 230]+0)/383;c3 = ([120 150 230]+128)/383;patch([0 1 1 0],[0 0 1 1],c1);patch([0 1 1 1-e 1-e 0+e],[0 0 1 1-e 0+e 0+e],c2);patch([0 0 1 1-e 0+e 0+e],[0 1 1 1-e 1-e 0+e],c3);plot([0 1 1 0 0],[0 0 1 1 0]);disp('Mux');
  dotprod{1..20} (20 alike) : neural/Weight Functions/dotprod
  "iz{1,1}" : Outport
      mask Display: e = 0.06;c1 = [120 230 180]/255;c2 = ([120 230 180]+0)/(256+128);c3 = ([120 230 180]+128)/(256+128);patch([0 1 1 0],[0 0 1 1],c1);patch([0 1 1 1-e 1-e 0+e],[0 0 1 1-e 0+e 0+e],c2);patch([0 0 1 1-e 0+e 0+e],[0 1 1 1-e 1-e 0+e],c3);plot([0 1 1 0 0],[0 0 1 1 0]);
  wires:
  "IW{1,1}(1,:)'"/1 -> dotprod1/1
  "pd{1,1}"/1 -> dotprod1/2, dotprod2/2, dotprod3/2, dotprod4/2, dotprod5/2, dotprod6/2, dotprod7/2, dotprod8/2, dotprod9/2, dotprod10/2, dotprod11/2, dotprod12/2, dotprod13/2, dotprod14/2, dotprod15/2, dotprod16/2, dotprod17/2, dotprod18/2, dotprod19/2, dotprod20/2
  dotprod1/1 -> Mux/1
  "IW{1,1}(2,:)'"/1 -> dotprod2/1
  dotprod2/1 -> Mux/2
  "IW{1,1}(3,:)'"/1 -> dotprod3/1
  dotprod3/1 -> Mux/3
  "IW{1,1}(4,:)'"/1 -> dotprod4/1
  dotprod4/1 -> Mux/4
  "IW{1,1}(5,:)'"/1 -> dotprod5/1
  dotprod5/1 -> Mux/5
  "IW{1,1}(6,:)'"/1 -> dotprod6/1
  dotprod6/1 -> Mux/6
  "IW{1,1}(7,:)'"/1 -> dotprod7/1
  dotprod7/1 -> Mux/7
  "IW{1,1}(8,:)'"/1 -> dotprod8/1
  dotprod8/1 -> Mux/8
  "IW{1,1}(9,:)'"/1 -> dotprod9/1
  dotprod9/1 -> Mux/9
  "IW{1,1}(10,:)'"/1 -> dotprod10/1
  dotprod10/1 -> Mux/10
  "IW{1,1}(11,:)'"/1 -> dotprod11/1
  dotprod11/1 -> Mux/11
  "IW{1,1}(12,:)'"/1 -> dotprod12/1
  dotprod12/1 -> Mux/12
  "IW{1,1}(13,:)'"/1 -> dotprod13/1
  dotprod13/1 -> Mux/13
  "IW{1,1}(14,:)'"/1 -> dotprod14/1
  dotprod14/1 -> Mux/14
  "IW{1,1}(15,:)'"/1 -> dotprod15/1
  dotprod15/1 -> Mux/15
  "IW{1,1}(16,:)'"/1 -> dotprod16/1
  dotprod16/1 -> Mux/16
  "IW{1,1}(17,:)'"/1 -> dotprod17/1
  dotprod17/1 -> Mux/17
  "IW{1,1}(18,:)'"/1 -> dotprod18/1
  dotprod18/1 -> Mux/18
  "IW{1,1}(19,:)'"/1 -> dotprod19/1
  dotprod19/1 -> Mux/19
  "IW{1,1}(20,:)'"/1 -> dotprod20/1
  dotprod20/1 -> Mux/20
  Mux/1 -> "iz{1,1}"/1

== system test_direct/Function Fitting Neural Network6/Layer 2/Delays 1 ==
  "p{2}" : Inport  PortDimensions=20
      mask Display: e = 0.06;c1 = [120 230 180]/255;c2 = ([120 230 180]+0)/(256+128);c3 = ([120 230 180]+128)/(256+128);patch([0 1 1 0],[0 0 1 1],c1);patch([0 1 1 1-e 1-e 0+e],[0 0 1 1-e 0+e 0+e],c2);patch([0 0 1 1-e 0+e 0+e],[0 1 1 1-e 1-e 0+e],c3);plot([0 1 1 0 0],[0 0 1 1 0]);
  mux : Mux  Inputs=1
      mask Display: e = 0.06;c1 = [120 150 230]/255;c2 = ([120 150 230]+0)/383;c3 = ([120 150 230]+128)/383;patch([0 1 1 0],[0 0 1 1],c1);patch([0 1 1 1-e 1-e 0+e],[0 0 1 1-e 0+e 0+e],c2);patch([0 0 1 1-e 0+e 0+e],[0 1 1 1-e 1-e 0+e],c3);plot([0 1 1 0 0],[0 0 1 1 0]);disp('Mux')
  "pd{2,1}" : Outport
      mask Display: e = 0.06;c1 = [120 230 180]/255;c2 = ([120 230 180]+0)/(256+128);c3 = ([120 230 180]+128)/(256+128);patch([0 1 1 0],[0 0 1 1],c1);patch([0 1 1 1-e 1-e 0+e],[0 0 1 1-e 0+e 0+e],c2);patch([0 0 1 1-e 0+e 0+e],[0 1 1 1-e 1-e 0+e],c3);plot([0 1 1 0 0],[0 0 1 1 0]);
  wires:
  "p{2}"/1 -> mux/1
  mux/1 -> "pd{2,1}"/1
